simulink model "ShowCaseModel"  (R2022b)
settings: Solver=VariableStepAuto  StartTime=0.0  StopTime=10  RelTol=1e-3
libraries: VACLib x6
settings Model: Creator=KarlO  LastModifiedBy=KarlO

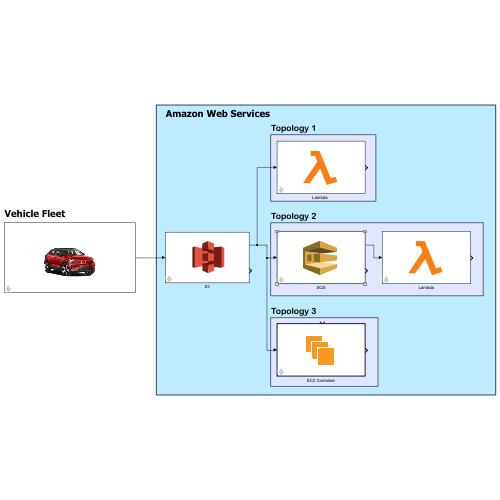
[thumbnail: Simulink's stored preview of the top-level diagram]
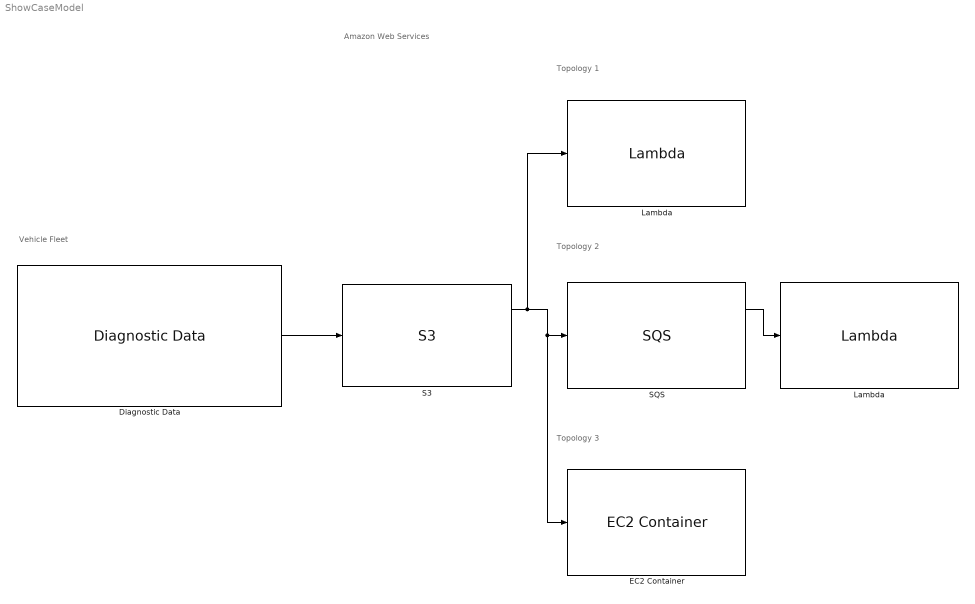
== system ShowCaseModel ==
  note: Topology 2
  note: Amazon Web Services
  note: Vehicle Fleet
  note: Topology 1
  note: Topology 3
  Diagnostic Data : VACLib/Vehicle Components/Diagnostic Data  cache_size=32  total_data_size=0  spurts=0
      settings: LibrarySourceBlock=|
      | simulink/User-Defined
      | Functions/MATLAB Function
  EC2 Container : VACLib/AWS Components/EC2 Container  no_cores=1  ram=8  no_instances=1
      settings: LibrarySourceBlock=|
      | simulink/User-Defined
      | Functions/MATLAB Function
  Lambda : VACLib/AWS Components/Lambda  parallel_instances=1  lambda_chunk_size=0
      settings: LibrarySourceBlock=|
      | simulink/User-Defined
      | Functions/MATLAB Function
  "Lambda  " : VACLib/AWS Components/Lambda  parallel_instances=1  lambda_chunk_size=0
      settings: LibrarySourceBlock=|
      | simulink/User-Defined
      | Functions/MATLAB Function
  S3 : VACLib/AWS Components/S3
      settings: LibrarySourceBlock=|
      | simulink/User-Defined
      | Functions/MATLAB Function
  SQS : VACLib/AWS Components/SQS  queue_size=32  timeout=0
      settings: LibrarySourceBlock=|
      | simulink/User-Defined
      | Functions/MATLAB Function
  wires:
  Diagnostic Data/1 -> S3/1
  S3/1 -> "Lambda  "/1, EC2 Container/1, SQS/1
  SQS/1 -> Lambda/1
